simulink model "hot_water_storage_tank"  (R2017a)
settings: Solver=VariableStepAuto  StartTime=0.0  StopTime=50000  RelTol=1e-3
settings Model: Creator=info  LastModifiedBy=admin

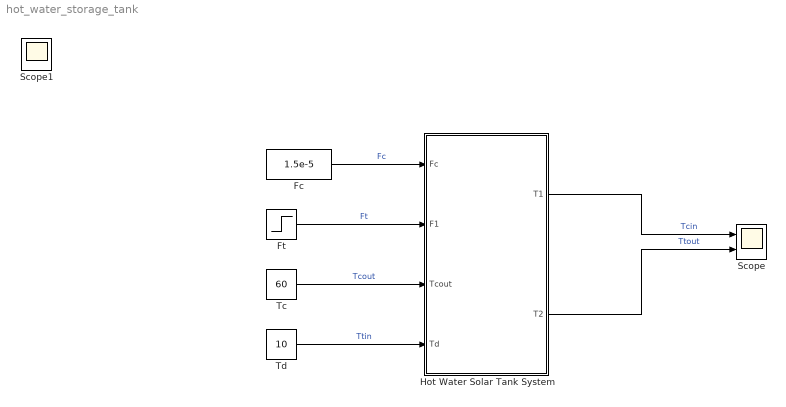
== system hot_water_storage_tank ==
  "Fc " : Constant  Value=1.5e-5
  "Ft " : Step  Time=0  After=1e-5  SampleTime=0
  Hot Water Solar Tank System : Subsystem
      mask Display: image('hot_water_tank.PNG');
  Scope : Scope  NumInputPorts=2
  Tc : Constant  Value=60
  Td : Constant  Value=10
  Scope1 : Scope
  wires:
  "Fc "/1 -> Hot Water Solar Tank System/1("Fc ")  "Fc"
  "Ft "/1 -> Hot Water Solar Tank System/2(F1)  "Ft"
  Tc/1 -> Hot Water Solar Tank System/3("Tcout ")  "Tcout"
  Td/1 -> Hot Water Solar Tank System/4("Td ")  "Ttin"
  Hot Water Solar Tank System/1("T1 ") -> Scope/1  "Tcin"
  Hot Water Solar Tank System/2("T2 ") -> Scope/2  "Ttout"

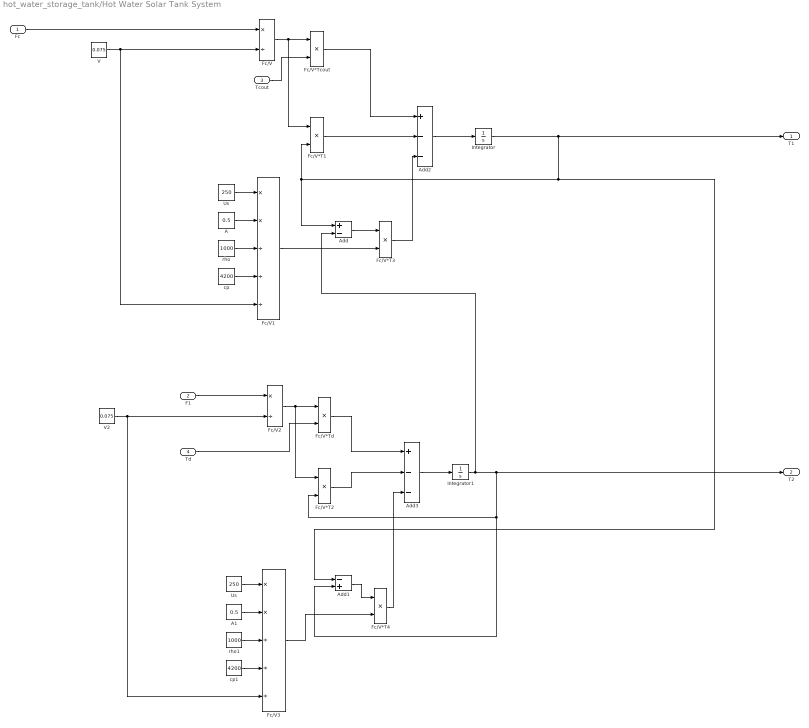
== system hot_water_storage_tank/Hot Water Solar Tank System ==
  "Fc " : Inport
  F1 : Inport  Port=2
  "Tcout " : Inport  Port=3
  "Td " : Inport  Port=4
  A : Constant  Value=0.5
  A1 : Constant  Value=0.5
  Add : Sum  Inputs=+-
  Add1 : Sum  Inputs=-+
  Add2 : Sum  Inputs=+--
  Add3 : Sum  Inputs=+--
  Fc/V : Product  Inputs=*/
  Fc/V*T{1..4} (4 alike) : Product  Inputs=**
  Fc/V*Tcout : Product  Inputs=**
  Fc/V*Td : Product  Inputs=**
  Fc/V1 : Product  Inputs=**///
  Fc/V2 : Product  Inputs=*/
  Fc/V3 : Product  Inputs=**///
  Integrator : Integrator  InitialCondition=16.87
  Integrator1 : Integrator  InitialCondition=10
  Us : Constant  Value=250
  "Us    " : Constant  Value=250
  V : Constant  Value=0.075
  V2 : Constant  Value=0.075
  cp : Constant  Value=4200
  cp1 : Constant  Value=4200
  rho : Constant  Value=1000
  rho1 : Constant  Value=1000
  "T1 " : Outport
  "T2 " : Outport  Port=2
  wires:
  V/1 -> Fc/V1/5, Fc/V/2
  "Us    "/1 -> Fc/V3/1
  Integrator1/1 -> Add1/2, Fc/V*T2/2, "T2 "/1, Add/2
  "Td "/1 -> Fc/V*Td/2
  "Fc "/1 -> Fc/V/1
  Fc/V/1 -> Fc/V*T1/1, Fc/V*Tcout/1
  rho/1 -> Fc/V1/3
  cp1/1 -> Fc/V3/4
  A1/1 -> Fc/V3/2
  Integrator/1 -> "T1 "/1, Add1/1, Fc/V*T1/2, Add/1
  Us/1 -> Fc/V1/1
  "Tcout "/1 -> Fc/V*Tcout/2
  rho1/1 -> Fc/V3/3
  Fc/V2/1 -> Fc/V*Td/1, Fc/V*T2/1
  V2/1 -> Fc/V2/2, Fc/V3/5
  F1/1 -> Fc/V2/1
  cp/1 -> Fc/V1/4
  A/1 -> Fc/V1/2
  Fc/V*Tcout/1 -> Add2/1
  Add2/1 -> Integrator/1
  Fc/V1/1 -> Fc/V*T3/2
  Fc/V*T3/1 -> Add2/3
  Fc/V*Td/1 -> Add3/1
  Add3/1 -> Integrator1/1
  Add/1 -> Fc/V*T3/1
  Fc/V*T1/1 -> Add2/2
  Fc/V*T2/1 -> Add3/2
  Fc/V*T4/1 -> Add3/3
  Fc/V3/1 -> Fc/V*T4/2
  Add1/1 -> Fc/V*T4/1
